simulink model "punto7"  (R2015a)
settings: Solver=ode45  StartTime=0.0  StopTime=10.0  RelTol=1e-3
settings Model: Creator=famu  LastModifiedBy=famu
settings DebuggingCC: UnderspecifiedInitializationDetection=Classic  MergeDetectMultiDrivingBlocksExec=none

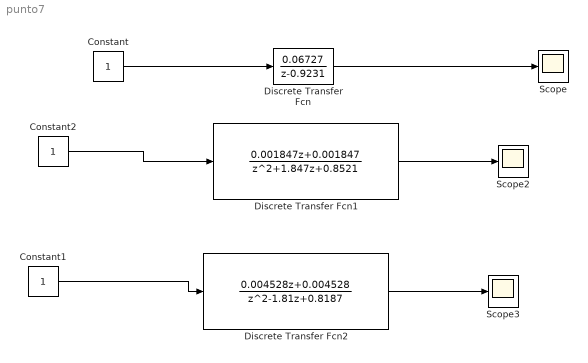
== system punto7 ==
  Constant : Constant
  Constant1 : Constant
  Constant2 : Constant
  Discrete Transfer Fcn : DiscreteTransferFcn  Numerator=[0 0.06727 ]  Denominator=[1 -0.9231]  SampleTime=0.01
  Discrete Transfer Fcn1 : DiscreteTransferFcn  Numerator=[0.001847 0.001847]  Denominator=[1 1.847 0.8521]  SampleTime=0.01
  Discrete Transfer Fcn2 : DiscreteTransferFcn  Numerator=[0.004528 0.004528]  Denominator="[1  -1.81 0.8187]"  SampleTime=0.01
  Scope : Scope
  Scope2 : Scope
      settings: SaveName=ScopeData2
  Scope3 : Scope
      settings: SaveName=ScopeData3
  wires:
  Discrete Transfer Fcn/1 -> Scope/1
  Constant/1 -> Discrete Transfer Fcn/1
  Discrete Transfer Fcn1/1 -> Scope2/1
  Constant2/1 -> Discrete Transfer Fcn1/1
  Constant1/1 -> Discrete Transfer Fcn2/1
  Discrete Transfer Fcn2/1 -> Scope3/1
